simulink model "ANN_and_Fuzzy_NCD"  (R2024a)
settings: Solver=ode23  StartTime=0.0  StopTime=200  RelTol=1e-8  EnableMultiTasking=on
model workspace (MAT data in the model file):
  targetSettings3.name = 'mapminmax'
  targetSettings3.xrows = 1
  targetSettings3.xmax = 42104.0119289
  targetSettings3.xmin = -1.27777923922
  targetSettings3.xrange = 42105.2897081
  targetSettings3.yrows = 1
  targetSettings3.ymax = 1
  targetSettings3.ymin = -1
  targetSettings3.yrange = 2
  targetSettings3.gain = 4.74999700481e-05
  targetSettings3.xoffset = -1.27777923922
  targetSettings3.no_change = 0
values from neighbouring files (symbols this model uses):
  I = in1'    [ann_training.m]
  T = out1'    [ann_training.m]
undefined symbols (not defined in the file or in its folder): B, DL, DQ, m, M, magnitude, rg, W, xb, xg, Xudot, yb, yg, Yvdot, zb, zg, Zwdot
libraries: neural x270, simulink x28, fuzblock x3
(part 1 of 12)
settings Model: Creator=hoang  LastModifiedBy=Long
settings SolverCC: ZeroCrossAlgorithm=Adaptive
settings DataIOCC: LimitDataPoints=on  SaveFormat=Array  SignalLoggingSaveFormat=ModelDataLogs  ReturnWorkspaceOutputs=off
settings OptimizationCC: InitFltsAndDblsToZero=on  LifeSpan=inf
settings DebuggingCC: SaveWithParameterizedLinksMsg=none  UnderspecifiedInitializationDetection=Classic  MergeDetectMultiDrivingBlocksExec=none  SignalResolutionControl=TryResolveAllWithWarning  IgnoredZcDiagnostic=none  SolverPrmCheckMsg=warning  MultiTaskDSMMsg=warning  MultiTaskCondExecSysMsg=none  UnconnectedInputMsg=warning  UnconnectedOutputMsg=warning  UnconnectedLineMsg=warning  SFUnexpectedBacktrackingDiag=warning  SFNoUnconditionalDefaultTransitionDiag=warning  SFExecutionAtInitializationDiag=none  ArithmeticOperatorsInVariantConditions=warning
settings HardwareCC: ProdBitPerPointer=32  ProdBitPerSizeT=32  ProdBitPerPtrDiffT=32  ProdLargestAtomicFloat=None  ProdIntDivRoundTo=Undefined  ProdEndianess=Unspecified  ProdWordSize=32  ProdHWDeviceType=32-bit Generic
settings ModelReferenceCC: EnableRefExpFcnMdlSchedulingChecks=on  PropagateSignalLabelsOutOfModel=off
settings RTWCC: GPUComputeCapability=3.5  DLArmComputeVersion=19.05
settings CodeAppCC: StateflowObjectComments=on
settings GRTTargetCC: TargetFcnLib=ansi_tfl_tmw.mat  TargetLangStandard=C89/C90 (ANSI)  CombineOutputUpdateFcns=off  GRTInterface=on
settings ConfigComp: CovMetricSettings=dw  CovSaveCumulativeToWorkspaceVar=on  CovSaveSingleToWorkspaceVar=on

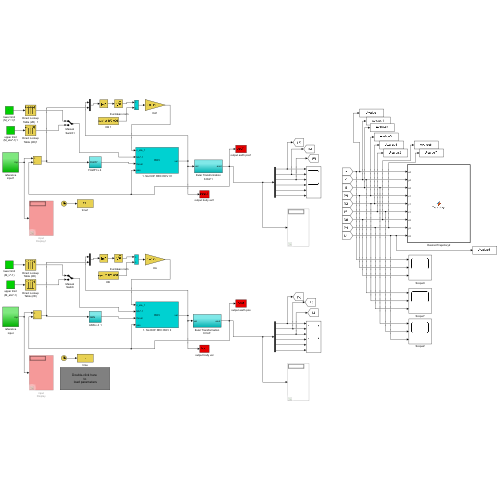
[thumbnail: Simulink's stored preview of the top-level diagram]
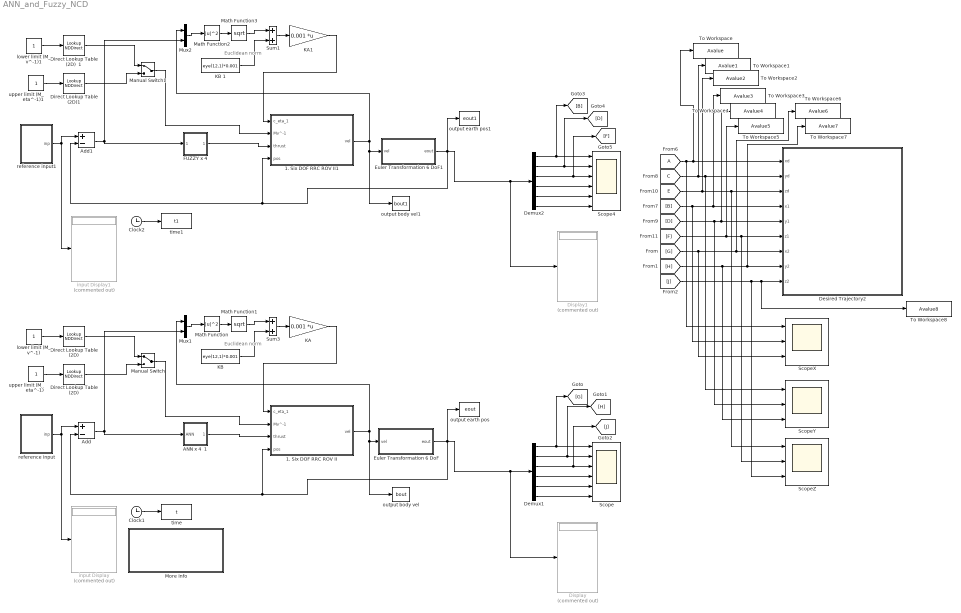
== system ANN_and_Fuzzy_NCD ==
  note: Euclidean norm
  note: Euclidean norm
  " ANN x 4  1" : Subsystem  AncestorBlock=|
      | rov_design_analysis/ROV Controller
      | Design
      | Applications/8. PID x 4
  " FUZZY x 4  " : Subsystem  AncestorBlock=|
      | rov_design_analysis/ROV Controller
      | Design
      | Applications/8. PID x 4
  1. Six DOF RRC ROV II : Subsystem  AncestorBlock=rov_design_analysis/ROV Models/1. Six DOF RRC ROV II
      mask Display: disp('ROV')
  1. Six DOF RRC ROV II1 : Subsystem  AncestorBlock=rov_design_analysis/ROV Models/1. Six DOF RRC ROV II
      mask Display: disp('ROV')
  Add : Sum  Inputs=+-
  Add1 : Sum  Inputs=+-
  Clock1 : Clock
  Clock2 : Clock
  Demux1 : Demux  Outputs=6
  Demux2 : Demux  Outputs=6
  Desired Trajectory2 : MATLAB Function  TreatAsAtomicUnit=on
  Direct Lookup Table (2D) : LookupNDDirect  InputsSelectThisObjectFromTable=Vector  Table=[0:0.1:1;0:0.1:1;0:0.1:1; 0:0.1:1 ; 0:0.1:1 ;0:0.1:1]*0.0001
  "Direct Lookup Table (2D)  " : LookupNDDirect  InputsSelectThisObjectFromTable=Vector  Table=-[0:0.1:1;0:0.1:1;0:0.1:1; 0:0.1:1 ; 0:0.1:1 ;0:0.1:1]*0.001
  Direct Lookup Table (2D)  1 : LookupNDDirect  InputsSelectThisObjectFromTable=Vector  Table=-[0:0.1:1;0:0.1:1;0:0.1:1; 0:0.1:1 ; 0:0.1:1 ;0:0.1:1]*0.001
  Direct Lookup Table (2D)1 : LookupNDDirect  InputsSelectThisObjectFromTable=Vector  Table=[0:0.1:1;0:0.1:1;0:0.1:1; 0:0.1:1 ; 0:0.1:1 ;0:0.1:1]*0.0001
  Display : Display  Commented=on
  Display1 : Display  Commented=on
  Euler Transformation 6 DoF : Subsystem  AncestorBlock=rov_design_analysis/Utilities/Euler Transformation 6 DoF
  Euler Transformation 6 DoF1 : Subsystem  AncestorBlock=rov_design_analysis/Utilities/Euler Transformation 6 DoF
  From6 : From  TagVisibility=global
  KA : Gain  Gain=0.001  Multiplication=Matrix(K*u)  SaturateOnIntegerOverflow=on  OutDataTypeStr=Inherit: Same as input  ParamDataTypeStr=Inherit: Same as input
  KA1 : Gain  Gain=0.001  Multiplication=Matrix(K*u)  SaturateOnIntegerOverflow=on  OutDataTypeStr=Inherit: Same as input  ParamDataTypeStr=Inherit: Same as input
  "KB " : Constant  Value=eye(12,1)*0.001
  KB 1 : Constant  Value=eye(12,1)*0.001
  Manual Switch : ManualSwitch
  Manual Switch1 : ManualSwitch
  Math Function : Math  Operator=magnitude^2  SignedPower=on
  Math Function1 : Math  Operator=sqrt  SignedPower=on
  Math Function2 : Math  Operator=magnitude^2  SignedPower=on
  Math Function3 : Math  Operator=sqrt  SignedPower=on
  More Info : Subsystem
      settings: OpenFcn=|
      | cd c:\Matlab7\toolbox\rov_design_analysis\\mat_file ;
      | load rrcrovf;
      | kp1=11;ki1=2;kd1=1; kp2=11;ki2=4;kd2=1;kp3=9;ki3=1;kd3=2;kp4=1;ki4=2;kd4=1;
      mask Display: disp('Double-click here \n to \n load parameters')
  Mux1 : Mux  Inputs=2
  Mux2 : Mux  Inputs=2
  Scope : Scope  NumInputPorts=6
  Scope4 : Scope  NumInputPorts=6
  ScopeX : Scope  NumInputPorts=3
  ScopeY : Scope  NumInputPorts=3
  ScopeZ : Scope  NumInputPorts=3
  Sum1 : Sum  OutDataTypeStr=double  SaturateOnIntegerOverflow=on
  Sum3 : Sum  OutDataTypeStr=double  SaturateOnIntegerOverflow=on
  To Workspace : ToWorkspace  VariableName=Avalue  SampleTime=-1
  To Workspace1 : ToWorkspace  VariableName=Avalue1  SampleTime=-1
  To Workspace2 : ToWorkspace  VariableName=Avalue2  SampleTime=-1
  To Workspace3 : ToWorkspace  VariableName=Avalue3  SampleTime=-1
  To Workspace4 : ToWorkspace  VariableName=Avalue4  SampleTime=-1
  To Workspace5 : ToWorkspace  VariableName=Avalue5  SampleTime=-1
  To Workspace6 : ToWorkspace  VariableName=Avalue6  SampleTime=-1
  To Workspace7 : ToWorkspace  VariableName=Avalue7  SampleTime=-1
  To Workspace8 : ToWorkspace  VariableName=Avalue8  SampleTime=-1
  input Display : Display  Commented=on
  input Display1 : Display  Commented=on
  lower limit (M_v^-1) : Constant
  lower limit (M_v^-1)1 : Constant
  output body vel : ToWorkspace  VariableName=bout  SampleTime=1
  output body vel1 : ToWorkspace  VariableName=bout1  SampleTime=1
  output earth pos : ToWorkspace  VariableName=eout  SampleTime=1
  output earth pos1 : ToWorkspace  VariableName=eout1  SampleTime=1
  reference input : Subsystem  AncestorBlock=|
      | rov_design_analysis/Scope
      | Utilities/pipe tracking
      | profile 
      | (Manual)
  reference input1 : Subsystem  AncestorBlock=|
      | rov_design_analysis/Scope
      | Utilities/pipe tracking
      | profile 
      | (Manual)
  time : ToWorkspace  VariableName=t  SampleTime=1
  time1 : ToWorkspace  VariableName=t1  SampleTime=1
  upper limit (M_eta^-1) : Constant
  upper limit (M_eta^-1)1 : Constant
  wires:
  Euler Transformation 6 DoF/1(eout) -> output earth pos/1, Add/2, 1. Six DOF RRC ROV II/4("pos "), Display/1, Demux1/1
  Clock1/1 -> time/1
  Add/1 -> " ANN x 4  1"/1(ANN), Mux1/2
  reference input/1(inp) -> Add/1, input Display/1
  1. Six DOF RRC ROV II/1(vel) -> output body vel/1, Euler Transformation 6 DoF/1(vel), Mux1/1
  upper limit (M_eta^-1)/1 -> Direct Lookup Table (2D)/1
  lower limit (M_v^-1)/1 -> "Direct Lookup Table (2D)  "/1
  "Direct Lookup Table (2D)  "/1 -> Manual Switch/1
  Manual Switch/1 -> 1. Six DOF RRC ROV II/2(Mv^-1)
  Direct Lookup Table (2D)/1 -> Manual Switch/2
  Sum3/1 -> KA/1
  "KB "/1 -> Sum3/2
  Mux1/1 -> Math Function/1
  Math Function/1 -> Math Function1/1
  Math Function1/1 -> Sum3/1
  KA/1 -> 1. Six DOF RRC ROV II/1(c_eta_1)
  Demux1/1 -> [G], Scope/1
  Demux1/2 -> [H], Scope/2
  Demux1/3 -> [J], Scope/3
  Demux1/6 -> Scope/6
  Demux1/5 -> Scope/5
  Demux1/4 -> Scope/4
  KB 1/1 -> Sum1/2
  Demux2/2 -> [D], Scope4/2
  [C] -> To Workspace1/1, ScopeY/1, Desired Trajectory2/2(yd)
  Sum1/1 -> KA1/1
  [D] -> ScopeY/2, To Workspace4/1, Desired Trajectory2/5(y1)
  lower limit (M_v^-1)1/1 -> Direct Lookup Table (2D)  1/1
  Manual Switch1/1 -> 1. Six DOF RRC ROV II1/2(Mv^-1)
  [F] -> To Workspace5/1, ScopeZ/2, Desired Trajectory2/6(z1)
  KA1/1 -> 1. Six DOF RRC ROV II1/1(c_eta_1)
  1. Six DOF RRC ROV II1/1(vel) -> output body vel1/1, Euler Transformation 6 DoF1/1(vel), Mux2/1
  From6/1 -> ScopeX/1, To Workspace/1, Desired Trajectory2/1(xd)
  Add1/1 -> Mux2/2, " FUZZY x 4  "/1(FUZZY)
  Demux2/4 -> Scope4/4
  Demux2/3 -> [F], Scope4/3
  Demux2/5 -> Scope4/5
  Demux2/6 -> Scope4/6
  Direct Lookup Table (2D)1/1 -> Manual Switch1/2
  Demux2/1 -> [B], Scope4/1
  reference input1/1(inp) -> Add1/1, input Display1/1
  Euler Transformation 6 DoF1/1(eout) -> output earth pos1/1, Add1/2, 1. Six DOF RRC ROV II1/4("pos "), Display1/1, Demux2/1
  Mux2/1 -> Math Function2/1
  Math Function2/1 -> Math Function3/1
  Math Function3/1 -> Sum1/1
  Direct Lookup Table (2D)  1/1 -> Manual Switch1/1
  upper limit (M_eta^-1)1/1 -> Direct Lookup Table (2D)1/1
  Clock2/1 -> time1/1
  [B] -> ScopeX/2, To Workspace3/1, Desired Trajectory2/4(x1)
  [E] -> ScopeZ/1, Desired Trajectory2/3(zd), To Workspace2/1
  " FUZZY x 4  "/1(" ") -> 1. Six DOF RRC ROV II1/3("thrust ")
  [G] -> ScopeX/3, To Workspace6/1, Desired Trajectory2/7(x2)
  [H] -> ScopeY/3, To Workspace7/1, Desired Trajectory2/8(y2)
  [J] -> ScopeZ/3, To Workspace8/1, Desired Trajectory2/9(z2)
  " ANN x 4  1"/1(" ") -> 1. Six DOF RRC ROV II/3("thrust ")

== system ANN_and_Fuzzy_NCD/ ANN x 4  1 ==
  ANN : Inport
  ANN X : Subsystem  Commented=on
      mask help: Feed-Forward Neural Network
      mask Display: e = 0.06;c1 = [120 150 230]/255;c2 = ([120 150 230]+0)/383;c3 = ([120 150 230]+128)/383;patch([0 1 1 0],[0 0 1 1],c1);patch([0 1 1 1-e 1-e 0+e],[0 0 1 1-e 0+e 0+e],c2);patch([0 0 1 1-e 0+e 0+e],[0 1 1 1-e 1-e 0+e],c3);plot([0 1 1 0 0],[0 0 1 1 0]);fprintf('NNET');port_label('input',1,' Input');port_label('output',1,'Output ');
  ANN Y : Subsystem  Commented=on
      mask help: Feed-Forward Neural Network
      mask Display: e = 0.06;c1 = [120 150 230]/255;c2 = ([120 150 230]+0)/383;c3 = ([120 150 230]+128)/383;patch([0 1 1 0],[0 0 1 1],c1);patch([0 1 1 1-e 1-e 0+e],[0 0 1 1-e 0+e 0+e],c2);patch([0 0 1 1-e 0+e 0+e],[0 1 1 1-e 1-e 0+e],c3);plot([0 1 1 0 0],[0 0 1 1 0]);fprintf('NNET');port_label('input',1,' Input');port_label('output',1,'Output ');
  ANN Z : Subsystem  Commented=on
      mask help: Feed-Forward Neural Network
      mask Display: e = 0.06;c1 = [120 150 230]/255;c2 = ([120 150 230]+0)/383;c3 = ([120 150 230]+128)/383;patch([0 1 1 0],[0 0 1 1],c1);patch([0 1 1 1-e 1-e 0+e],[0 0 1 1-e 0+e 0+e],c2);patch([0 0 1 1-e 0+e 0+e],[0 1 1 1-e 1-e 0+e],c3);plot([0 1 1 0 0],[0 0 1 1 0]);fprintf('NNET');port_label('input',1,' Input');port_label('output',1,'Output ');
  Demux1 : Demux  Outputs=6
      settings: DisplayOption=none
  Mux2 : Mux  Inputs=6
  Subsystem : Subsystem
  Subsystem1 : Subsystem
  Subsystem2 : Subsystem
  X_1 : Subsystem
      mask help: Feed-Forward Neural Network
      mask Display: e = 0.06;c1 = [120 150 230]/255;c2 = ([120 150 230]+0)/383;c3 = ([120 150 230]+128)/383;patch([0 1 1 0],[0 0 1 1],c1);patch([0 1 1 1-e 1-e 0+e],[0 0 1 1-e 0+e 0+e],c2);patch([0 0 1 1-e 0+e 0+e],[0 1 1 1-e 1-e 0+e],c3);plot([0 1 1 0 0],[0 0 1 1 0]);fprintf('NNET');port_label('input',1,' Input');port_label('output',1,'Output ');
  Y_1 : Subsystem
      mask help: Feed-Forward Neural Network
      mask Display: e = 0.06;c1 = [120 150 230]/255;c2 = ([120 150 230]+0)/383;c3 = ([120 150 230]+128)/383;patch([0 1 1 0],[0 0 1 1],c1);patch([0 1 1 1-e 1-e 0+e],[0 0 1 1-e 0+e 0+e],c2);patch([0 0 1 1-e 0+e 0+e],[0 1 1 1-e 1-e 0+e],c3);plot([0 1 1 0 0],[0 0 1 1 0]);fprintf('NNET');port_label('input',1,' Input');port_label('output',1,'Output ');
  Z_1 : Subsystem
      mask help: Feed-Forward Neural Network
      mask Display: e = 0.06;c1 = [120 150 230]/255;c2 = ([120 150 230]+0)/383;c3 = ([120 150 230]+128)/383;patch([0 1 1 0],[0 0 1 1],c1);patch([0 1 1 1-e 1-e 0+e],[0 0 1 1-e 0+e 0+e],c2);patch([0 0 1 1-e 0+e 0+e],[0 1 1 1-e 1-e 0+e],c3);plot([0 1 1 0 0],[0 0 1 1 0]);fprintf('NNET');port_label('input',1,' Input');port_label('output',1,'Output ');
  " " : Outport
  wires:
  Demux1/4 -> Mux2/4
  Demux1/5 -> Mux2/5
  Demux1/6 -> Mux2/6
  Demux1/2 -> Subsystem1/1(In1)
  Demux1/3 -> Subsystem2/1(In1)
  ANN/1 -> Demux1/1
  Mux2/1 -> " "/1
  Demux1/1 -> Subsystem/1(In1)
  Subsystem/1(Out1) -> X_1/1(Input)
  Subsystem1/1(Out1) -> Y_1/1(Input)
  Subsystem2/1(Out1) -> Z_1/1(Input)
  X_1/1(Output) -> Mux2/1
  Z_1/1(Output) -> Mux2/3
  Y_1/1(Output) -> Mux2/2

== system ANN_and_Fuzzy_NCD/ FUZZY x 4   ==
  FUZZY : Inport
  Demux1 : Demux  Outputs=6
      settings: DisplayOption=none
  Mux2 : Mux  Inputs=6
  Subsystem1 : Subsystem
  Subsystem5 : Subsystem
  Subsystem6 : Subsystem
  " " : Outport
  wires:
  Demux1/1 -> Subsystem1/1(Error)
  Demux1/4 -> Mux2/4
  Demux1/5 -> Mux2/5
  Subsystem1/1(Output) -> Mux2/1
  Subsystem6/1(Output) -> Mux2/3
  Demux1/2 -> Subsystem5/1(Error)
  Subsystem5/1(Output) -> Mux2/2
  Demux1/3 -> Subsystem6/1(Error)
  FUZZY/1 -> Demux1/1
  Mux2/1 -> " "/1
  Demux1/6 -> Mux2/6

== system ANN_and_Fuzzy_NCD/1. Six DOF RRC ROV II ==
  c_eta_1 : Inport
  Mv^-1 : Inport  Port=2
  "thrust " : Inport  Port=3
  "pos " : Inport  Port=4
  Centripetal & Coriolis : Subsystem
      mask Display: disp('Coriolis \n& Centrpetal \nMatrix')
  Demux : Demux  Outputs=2
  Hydrodynamic Damping : Subsystem
      mask Display: disp('Hydrodynamic \nDamping')
  Integrator1 : Integrator  UpperSaturationLimit=5  LowerSaturationLimit=1
  Mass Inertia Matrix : Subsystem
      mask Display: disp('Inverse Mass \n Inertia \n Matrix')
  Pseudo Inverse : Gain  Gain=pinv(T)  Multiplication=Matrix(K*u)  SaturateOnIntegerOverflow=on  OutDataTypeStr=Inherit: Same as input  ParamDataTypeStr=Inherit: Same as input
  Restoring Forces : Subsystem
      mask Display: disp('Restoring\nForce')
  Sum1 : Sum  Inputs=+---  OutDataTypeStr=double  SaturateOnIntegerOverflow=on
  Sum2 : Sum  OutDataTypeStr=double  SaturateOnIntegerOverflow=on
  Sum3 : Sum  OutDataTypeStr=double  SaturateOnIntegerOverflow=on
  Sum4 : Sum  OutDataTypeStr=double  SaturateOnIntegerOverflow=on
  Thruster Configuration Matrix (n X n) : Subsystem  AncestorBlock=|  mask(Thruster Configuration Matrix){T=T}
      | rov_design_analysis/ROV
      | Models/4.  Thruster Configuration Matrix
      | (n X n)
      mask prompts: T "Insert Thruster Configuration Matrix"
      mask help: Provide the thruster configuration matrix using summation of forces and moment about the vehicle's C.G.
      mask Display: disp('Thruster \n Configuration')
  vel : Outport
  wires:
  Sum1/1 -> Mass Inertia Matrix/1(In)
  "pos "/1 -> Restoring Forces/1(pos)
  Restoring Forces/1(gravitational force) -> Sum1/2
  "thrust "/1 -> Pseudo Inverse/1
  Pseudo Inverse/1 -> Thruster Configuration Matrix (n X n)/1(In1)
  Sum2/1 -> Integrator1/1
  Mass Inertia Matrix/1(Out) -> Sum2/2
  Mv^-1/1 -> Sum2/1
  Centripetal & Coriolis/1(force) -> Sum3/2
  Sum3/1 -> Sum1/4
  Sum4/1 -> Sum1/3
  Hydrodynamic Damping/1(damping force) -> Sum4/2
  c_eta_1/1 -> Demux/1
  Demux/2 -> Sum4/1
  Demux/1 -> Sum3/1
  Integrator1/1 -> vel/1, Centripetal & Coriolis/1(vel), Hydrodynamic Damping/1(vel)
  Thruster Configuration Matrix (n X n)/1(Out1) -> Sum1/1

== system ANN_and_Fuzzy_NCD/1. Six DOF RRC ROV II1 ==
  c_eta_1 : Inport
  Mv^-1 : Inport  Port=2
  "thrust " : Inport  Port=3
  "pos " : Inport  Port=4
  Centripetal & Coriolis : Subsystem
      mask Display: disp('Coriolis \n& Centrpetal \nMatrix')
  Demux : Demux  Outputs=2
  Hydrodynamic Damping : Subsystem
      mask Display: disp('Hydrodynamic \nDamping')
  Integrator1 : Integrator  UpperSaturationLimit=5  LowerSaturationLimit=1
  Mass Inertia Matrix : Subsystem
      mask Display: disp('Inverse Mass \n Inertia \n Matrix')
  Pseudo Inverse : Gain  Gain=pinv(T)  Multiplication=Matrix(K*u)  SaturateOnIntegerOverflow=on  OutDataTypeStr=Inherit: Same as input  ParamDataTypeStr=Inherit: Same as input
  Restoring Forces : Subsystem
      mask Display: disp('Restoring\nForce')
  Sum1 : Sum  Inputs=+---  OutDataTypeStr=double  SaturateOnIntegerOverflow=on
  Sum2 : Sum  OutDataTypeStr=double  SaturateOnIntegerOverflow=on
  Sum3 : Sum  OutDataTypeStr=double  SaturateOnIntegerOverflow=on
  Sum4 : Sum  OutDataTypeStr=double  SaturateOnIntegerOverflow=on
  Thruster Configuration Matrix (n X n) : Subsystem  AncestorBlock=|  mask(Thruster Configuration Matrix){T=T}
      | rov_design_analysis/ROV
      | Models/4.  Thruster Configuration Matrix
      | (n X n)
      mask prompts: T "Insert Thruster Configuration Matrix"
      mask help: Provide the thruster configuration matrix using summation of forces and moment about the vehicle's C.G.
      mask Display: disp('Thruster \n Configuration')
  vel : Outport
  wires:
  Sum1/1 -> Mass Inertia Matrix/1(In)
  "pos "/1 -> Restoring Forces/1(pos)
  Restoring Forces/1(gravitational force) -> Sum1/2
  Thruster Configuration Matrix (n X n)/1(Out1) -> Sum1/1
  "thrust "/1 -> Pseudo Inverse/1
  Pseudo Inverse/1 -> Thruster Configuration Matrix (n X n)/1(In1)
  Sum2/1 -> Integrator1/1
  Integrator1/1 -> vel/1, Centripetal & Coriolis/1(vel), Hydrodynamic Damping/1(vel)
  Mass Inertia Matrix/1(Out) -> Sum2/2
  Mv^-1/1 -> Sum2/1
  Centripetal & Coriolis/1(force) -> Sum3/2
  Sum3/1 -> Sum1/4
  Sum4/1 -> Sum1/3
  Hydrodynamic Damping/1(damping force) -> Sum4/2
  c_eta_1/1 -> Demux/1
  Demux/2 -> Sum4/1
  Demux/1 -> Sum3/1

== system ANN_and_Fuzzy_NCD/Euler Transformation 6 DoF ==
  vel : Inport
  Demux : Demux  Outputs=2
      settings: DisplayOption=none
  Demux1 : Demux  Outputs=2
      settings: DisplayOption=none
  Environment Impact2 : Subsystem
  Intregrator2 : Integrator
  Mux1 : Mux  Inputs=2
  Sum : Sum  Inputs=|++
  Terminator : Terminator
  Transformation matrix R : Subsystem
      mask Display: disp('Transformation R')
  Transformation matrix T : Subsystem
      mask Display: disp('Transformation T')
  eout : Outport  InitialOutput=0
  wires:
  Mux1/1 -> Intregrator2/1
  Intregrator2/1 -> Sum/2, Demux1/1
  Demux/2 -> Transformation matrix R/1(angular body velocity)
  Demux/1 -> Transformation matrix T/1(translational body velocity)
  vel/1 -> Demux/1
  Demux1/2 -> Transformation matrix T/2(angular position), Transformation matrix R/2(angular position)
  Transformation matrix R/1(angular earth velocity) -> Mux1/2
  Transformation matrix T/1(translational earth velocity) -> Mux1/1
  Demux1/1 -> Terminator/1
  Sum/1 -> eout/1
  Environment Impact2/1(F_current) -> Sum/1

== system ANN_and_Fuzzy_NCD/Euler Transformation 6 DoF1 ==
  vel : Inport
  Demux : Demux  Outputs=2
      settings: DisplayOption=none
  Demux1 : Demux  Outputs=2
      settings: DisplayOption=none
  Environment Impact2 : Subsystem
  Intregrator2 : Integrator
  Mux1 : Mux  Inputs=2
  Sum : Sum  Inputs=|++
  Terminator : Terminator
  Transformation matrix R : Subsystem
      mask Display: disp('Transformation R')
  Transformation matrix T : Subsystem
      mask Display: disp('Transformation T')
  eout : Outport  InitialOutput=0
  wires:
  Mux1/1 -> Intregrator2/1
  Intregrator2/1 -> Sum/2, Demux1/1
  Demux/2 -> Transformation matrix R/1(angular body velocity)
  Demux/1 -> Transformation matrix T/1(translational body velocity)
  vel/1 -> Demux/1
  Demux1/2 -> Transformation matrix T/2(angular position), Transformation matrix R/2(angular position)
  Transformation matrix R/1(angular earth velocity) -> Mux1/2
  Transformation matrix T/1(translational earth velocity) -> Mux1/1
  Demux1/1 -> Terminator/1
  Sum/1 -> eout/1
  Environment Impact2/1(F_current) -> Sum/1

== system ANN_and_Fuzzy_NCD/More Info ==

== system ANN_and_Fuzzy_NCD/reference input ==
  Goto : Goto  TagVisibility=global
  Ground : Ground
  Mux : Mux  Inputs=6
  Repeating Sequence Stair13 : simulink/Sources/Repeating Sequence Stair  OutValues="[0 1 2 3 4 5 6 7 8 9 10 11 12 13 14 15 16 17 18 19 20 20 20 20 20 20 20 20 20 20 20 20 20 20 20 20 20 20 20 20 20 20 20 20 20 20 20 20 20 20 20 20 20 20 20 20 20 20 20 20 20 20 20 20 20 20 20 20 20 20 20 20 20 20 20 20 20 20 20 20 20 20 20 20 20 20 20 20 20 20 20 20 20 20 20 20   ].'"  tsamp=2.5  OutMin=[]  OutMax=[]  OutDataTypeStr=double  OutputDataTypeScalingMode=double  OutDataType=fixdt(0,8)  ConRadixGroup=Best Precision: Vector-wise  OutScaling=2^-12
  Repeating Sequence Stair14 : simulink/Sources/Repeating Sequence Stair  OutValues="[0 0.5 1 1.5 2 2.5 3 3.5 4 4.5 5 5.5 6 6.5 7 7.5 8 8.5 9 9.5 10 10 10 10 10 10 10 10 10 10 10 10 10 10 10 10 10 10 10 10 10 10 10 10 10 10 10 10 10 10 10 10 10 10 10 10 10 10 10 10 10 10 10 10 10 10 10 10 10 10 10 10 10 10 10 10 10 10 10 10 10 10 10 10 10 10 10 10 10 10 10 10 10 10 10 10 10 10 10 10 10 10 10 10 10 10 10 10 10 10 10 10 10 10 10 10 10 10 10 10 10 10 10 10 10 10 10 10 10 10 10 10 10 10 10 10 10 10 10 10 10 10 10 10 10 10 10 10 10 10 10 10 10 10 10 10 10 10 10 10 10 10 10 10 10 10 10 10 10 10 10 10 10     ].'"  tsamp=2.5  OutMin=[]  OutMax=[]  OutDataTypeStr=double  OutputDataTypeScalingMode=double  OutDataType=fixdt(0,8)  ConRadixGroup=Best Precision: Vector-wise  OutScaling=2^-12
  Repeating Sequence Stair15 : simulink/Sources/Repeating Sequence Stair  OutValues="[0 1 2 3 4 5 6 7 8 9 10 11 12 13 14 15 16 17 18 19 20 20 20 20 20 20 20 20 20 20 20 20 20 20 20 20 20 20 20 20 20 20 20 20 20 20 20 20 20 20 20 20 20 20 20 20 20 20 20 20 20 20 20 20 20 20 20 20 20 20 20 20 20 20 20 20 20 20 20 20 20 20 20 20 20    ].'"  tsamp=2.5  OutMin=[]  OutMax=[]  OutDataTypeStr=double  OutputDataTypeScalingMode=double  OutDataType=fixdt(0,8)  ConRadixGroup=Best Precision: Vector-wise  OutScaling=2^-12
  Repeating Sequence Stair3 : simulink/Sources/Repeating Sequence Stair  OutValues="[0 0 0 0 0 0 0 0 0 0 0 0 0 0 0 0 0 0 0 0 0 0 0 0 0 0 0 0 0 0 0 0 0 0 0 0 0 0 0 0 0 0 0 0 0 0 0 0 0 0 0 0 0 0 0 0 0 0 0 0 0 0 0 0 0 0 0 0 0 0 0 0 0 0 0 0 0 0 0 0 0 0 0 0 0 0 0 0 0 0 0 0 0 0 0 0 0 0 0 0 0 0 0 0 0 0 0 0 0 0 0 0 0 0 0 0 0 0 0 0 0 0 0 0 0 0 0 0 0 0 0 0 0 0 0 0 0 0 0 0 0 0 0 0 0 0 0 0 0 0 0 0 0 0 0 0 0 0 0 0 0 0 0 0 0  ].'"  tsamp=2.5  OutMin=[]  OutMax=[]  OutDataTypeStr=double  OutputDataTypeScalingMode=double  OutDataType=fixdt(0,8)  ConRadixGroup=Best Precision: Vector-wise  OutScaling=2^-12
  Repeating Sequence Stair4 : simulink/Sources/Repeating Sequence Stair  Commented=on  OutValues="[0 1 2 3 4 5 6 7 8 9 10 10 10 10 10 10 10 10 10 10 10 10 10 10 10 10 10 10 10 10 10 11 12 13 14 15 16 17 18 19 20 20 20 20 20 20 20 20 20 20 20 19 18 17 16 15 14 13 12 11 10 10 10 10 10 10 10 10 10 10 10 10 10 10 10 10 10 10 10 10 10 10 10 10 10 10 10 10 10 10 10 10 10 10 10 10 10 10 10 10  ].'"  tsamp=2.5  OutMin=[]  OutMax=[]  OutDataTypeStr=double  OutputDataTypeScalingMode=double  OutDataType=fixdt(0,8)  ConRadixGroup=Best Precision: Vector-wise  OutScaling=2^-12
  Repeating Sequence Stair5 : simulink/Sources/Repeating Sequence Stair  Commented=on  OutValues=[0 0 0 0 0 0 0 0 0 0 0 0.5 1 1.5 2 2.5 3 3.5 4 4.5 5 5 5 5 5 5 5 5 5 5 5 5 5 5 5 5 5 5 5 5 5 5.5 6 6.5 7 7.5 8 8.5 9 9.5 10 10 10 10 10 10 10 10 10 10 10 10 10 10 10 10 10 10 10 10 10 10 10 10 10 10 10 10 10 10 10 10 10 10 10 10 10 10 10 10 10 10 10 10 10 10 10 10 10 10 10 10 10 10 10 10 10 10 10 10 10 10 10 10 10 10 10 10 10 10 10 10 10 10 10 10].'  tsamp=2.5  OutMin=[]  OutMax=[]  OutDataTypeStr=double  OutputDataTypeScalingMode=double  OutDataType=fixdt(0,8)  ConRadixGroup=Best Precision: Vector-wise  OutScaling=2^-12
  Repeating Sequence Stair6 : simulink/Sources/Repeating Sequence Stair  Commented=on  OutValues="[0 0 0 0 0 0 0 0 0 0 0 0 0 0 0 0 0 0 0 0 0 1 2 3 4 5 6 7 8 9 10 10 10 10 10 10 10 10 10 10 10 10 10 10 10 10 10 10 10 10 10 10 10 10 10 10 10 10 10 10 10 10 10 10 10 10 10 10 10 10 10 10 10 10 10 10 10 10 10 10 10 10 10 10 10 10 10 10 10 10 10 10 10 10 10 10 10 10 10 10 10 10 10 10 10 10 10 10 10 10 10 10 10 10 10 10 10 10 10 10 10 10 10 10 10 10 10 10 10 10 10 10 10 10  ].'"  tsamp=2.5  OutMin=[]  OutMax=[]  OutDataTypeStr=double  OutputDataTypeScalingMode=double  OutDataType=fixdt(0,8)  ConRadixGroup=Best Precision: Vector-wise  OutScaling=2^-12
  inp : Outport
  tag scope: C=global, E=global
  wires:
  Mux/1 -> inp/1
  Ground/1 -> Mux/4, Mux/5
  Repeating Sequence Stair3/1 -> Mux/6
  Repeating Sequence Stair13/1 -> Goto/1, Mux/1
  Repeating Sequence Stair14/1 -> [C], Mux/2
  Repeating Sequence Stair15/1 -> [E], Mux/3

== system ANN_and_Fuzzy_NCD/reference input1 ==
  Ground : Ground
  Mux : Mux  Inputs=6
  Repeating Sequence Stair13 : simulink/Sources/Repeating Sequence Stair  OutValues="[0 1 2 3 4 5 6 7 8 9 10 11 12 13 14 15 16 17 18 19 20 20 20 20 20 20 20 20 20 20 20 20 20 20 20 20 20 20 20 20 20 20 20 20 20 20 20 20 20 20 20 20 20 20 20 20 20 20 20 20 20 20 20 20 20 20 20 20 20 20 20 20 20 20 20 20 20 20 20 20 20 20 20 20 20 20 20 20 20 20 20 20 20 20 20 20   ].'"  tsamp=2.5  OutMin=[]  OutMax=[]  OutDataTypeStr=double  OutputDataTypeScalingMode=double  OutDataType=fixdt(0,8)  ConRadixGroup=Best Precision: Vector-wise  OutScaling=2^-12
  Repeating Sequence Stair14 : simulink/Sources/Repeating Sequence Stair  OutValues="[0 0.5 1 1.5 2 2.5 3 3.5 4 4.5 5 5.5 6 6.5 7 7.5 8 8.5 9 9.5 10 10 10 10 10 10 10 10 10 10 10 10 10 10 10 10 10 10 10 10 10 10 10 10 10 10 10 10 10 10 10 10 10 10 10 10 10 10 10 10 10 10 10 10 10 10 10 10 10 10 10 10 10 10 10 10 10 10 10 10 10 10 10 10 10 10 10 10 10 10 10 10 10 10 10 10 10 10 10 10 10 10 10 10 10 10 10 10 10 10 10 10 10 10 10 10 10 10 10 10 10 10 10 10 10 10 10 10 10 10 10 10 10 10 10 10 10 10 10 10 10 10 10 10 10 10 10 10 10 10 10 10 10 10 10 10 10 10 10 10 10 10 10 10 10 10 10 10 10 10 10 10 10     ].'"  tsamp=2.5  OutMin=[]  OutMax=[]  OutDataTypeStr=double  OutputDataTypeScalingMode=double  OutDataType=fixdt(0,8)  ConRadixGroup=Best Precision: Vector-wise  OutScaling=2^-12
  Repeating Sequence Stair15 : simulink/Sources/Repeating Sequence Stair  OutValues="[0 1 2 3 4 5 6 7 8 9 10 11 12 13 14 15 16 17 18 19 20 20 20 20 20 20 20 20 20 20 20 20 20 20 20 20 20 20 20 20 20 20 20 20 20 20 20 20 20 20 20 20 20 20 20 20 20 20 20 20 20 20 20 20 20 20 20 20 20 20 20 20 20 20 20 20 20 20 20 20 20 20 20 20 20    ].'"  tsamp=2.5  OutMin=[]  OutMax=[]  OutDataTypeStr=double  OutputDataTypeScalingMode=double  OutDataType=fixdt(0,8)  ConRadixGroup=Best Precision: Vector-wise  OutScaling=2^-12
  Repeating Sequence Stair3 : simulink/Sources/Repeating Sequence Stair  OutValues="[0 0 0 0 0 0 0 0 0 0 0 0 0 0 0 0 0 0 0 0 0 0 0 0 0 0 0 0 0 0 0 0 0 0 0 0 0 0 0 0 0 0 0 0 0 0 0 0 0 0 0 0 0 0 0 0 0 0 0 0 0 0 0 0 0 0 0 0 0 0 0 0 0 0 0 0 0 0 0 0 0 0 0 0 0 0 0 0 0 0 0 0 0 0 0 0 0 0 0 0 0 0 0 0 0 0 0 0 0 0 0 0 0 0 0 0 0 0 0 0 0 0 0 0 0 0 0 0 0 0 0 0 0 0 0 0 0 0 0 0 0 0 0 0 0 0 0 0 0 0 0 0 0 0 0 0 0 0 0 0 0 0 0 0 0  ].'"  tsamp=2.5  OutMin=[]  OutMax=[]  OutDataTypeStr=double  OutputDataTypeScalingMode=double  OutDataType=fixdt(0,8)  ConRadixGroup=Best Precision: Vector-wise  OutScaling=2^-12
  Repeating Sequence Stair4 : simulink/Sources/Repeating Sequence Stair  Commented=on  OutValues="[0 1 2 3 4 5 6 7 8 9 10 10 10 10 10 10 10 10 10 10 10 10 10 10 10 10 10 10 10 10 10 11 12 13 14 15 16 17 18 19 20 20 20 20 20 20 20 20 20 20 20 19 18 17 16 15 14 13 12 11 10 10 10 10 10 10 10 10 10 10 10 10 10 10 10 10 10 10 10 10 10 10 10 10 10 10 10 10 10 10 10 10 10 10 10 10 10 10 10 10  ].'"  tsamp=2.5  OutMin=[]  OutMax=[]  OutDataTypeStr=double  OutputDataTypeScalingMode=double  OutDataType=fixdt(0,8)  ConRadixGroup=Best Precision: Vector-wise  OutScaling=2^-12
  Repeating Sequence Stair5 : simulink/Sources/Repeating Sequence Stair  Commented=on  OutValues=[0 0 0 0 0 0 0 0 0 0 0 0.5 1 1.5 2 2.5 3 3.5 4 4.5 5 5 5 5 5 5 5 5 5 5 5 5 5 5 5 5 5 5 5 5 5 5.5 6 6.5 7 7.5 8 8.5 9 9.5 10 10 10 10 10 10 10 10 10 10 10 10 10 10 10 10 10 10 10 10 10 10 10 10 10 10 10 10 10 10 10 10 10 10 10 10 10 10 10 10 10 10 10 10 10 10 10 10 10 10 10 10 10 10 10 10 10 10 10 10 10 10 10 10 10 10 10 10 10 10 10 10 10 10 10 10].'  tsamp=2.5  OutMin=[]  OutMax=[]  OutDataTypeStr=double  OutputDataTypeScalingMode=double  OutDataType=fixdt(0,8)  ConRadixGroup=Best Precision: Vector-wise  OutScaling=2^-12
  Repeating Sequence Stair6 : simulink/Sources/Repeating Sequence Stair  Commented=on  OutValues="[0 0 0 0 0 0 0 0 0 0 0 0 0 0 0 0 0 0 0 0 0 1 2 3 4 5 6 7 8 9 10 10 10 10 10 10 10 10 10 10 10 10 10 10 10 10 10 10 10 10 10 10 10 10 10 10 10 10 10 10 10 10 10 10 10 10 10 10 10 10 10 10 10 10 10 10 10 10 10 10 10 10 10 10 10 10 10 10 10 10 10 10 10 10 10 10 10 10 10 10 10 10 10 10 10 10 10 10 10 10 10 10 10 10 10 10 10 10 10 10 10 10 10 10 10 10 10 10 10 10 10 10 10 10  ].'"  tsamp=2.5  OutMin=[]  OutMax=[]  OutDataTypeStr=double  OutputDataTypeScalingMode=double  OutDataType=fixdt(0,8)  ConRadixGroup=Best Precision: Vector-wise  OutScaling=2^-12
  inp : Outport
  wires:
  Mux/1 -> inp/1
  Repeating Sequence Stair3/1 -> Mux/6
  Ground/1 -> Mux/4, Mux/5
  Repeating Sequence Stair13/1 -> Mux/1
  Repeating Sequence Stair14/1 -> Mux/2
  Repeating Sequence Stair15/1 -> Mux/3

== system ANN_and_Fuzzy_NCD/ ANN x 4  1/ANN X ==
  Input : Inport  PortDimensions=2
      mask Display: e = 0.06;c1 = [120 230 180]/255;c2 = ([120 230 180]+0)/(256+128);c3 = ([120 230 180]+128)/(256+128);patch([0 1 1 0],[0 0 1 1],c1);patch([0 1 1 1-e 1-e 0+e],[0 0 1 1-e 0+e 0+e],c2);patch([0 0 1 1-e 0+e 0+e],[0 1 1 1-e 1-e 0+e],c3);plot([0 1 1 0 0],[0 0 1 1 0]);
  Layer 1 : Subsystem
      mask Display: e = 0.06;c1 = [120 150 230]/255;c2 = ([120 150 230]+0)/383;c3 = ([120 150 230]+128)/383;patch([0 1 1 0],[0 0 1 1],c1);patch([0 1 1 1-e 1-e 0+e],[0 0 1 1-e 0+e 0+e],c2);patch([0 0 1 1-e 0+e 0+e],[0 1 1 1-e 1-e 0+e],c3);plot([0 1 1 0 0],[0 0 1 1 0]);
  Layer 2 : Subsystem
      mask Display: e = 0.06;c1 = [120 150 230]/255;c2 = ([120 150 230]+0)/383;c3 = ([120 150 230]+128)/383;patch([0 1 1 0],[0 0 1 1],c1);patch([0 1 1 1-e 1-e 0+e],[0 0 1 1-e 0+e 0+e],c2);patch([0 0 1 1-e 0+e 0+e],[0 1 1 1-e 1-e 0+e],c3);plot([0 1 1 0 0],[0 0 1 1 0]);
  Layer 3 : Subsystem
      mask Display: e = 0.06;c1 = [120 150 230]/255;c2 = ([120 150 230]+0)/383;c3 = ([120 150 230]+128)/383;patch([0 1 1 0],[0 0 1 1],c1);patch([0 1 1 1-e 1-e 0+e],[0 0 1 1-e 0+e 0+e],c2);patch([0 0 1 1-e 0+e 0+e],[0 1 1 1-e 1-e 0+e],c3);plot([0 1 1 0 0],[0 0 1 1 0]);
  Process Input 1 : Subsystem
      mask Display: e = 0.06;c1 = [120 150 230]/255;c2 = ([120 150 230]+0)/383;c3 = ([120 150 230]+128)/383;patch([0 1 1 0],[0 0 1 1],c1);patch([0 1 1 1-e 1-e 0+e],[0 0 1 1-e 0+e 0+e],c2);patch([0 0 1 1-e 0+e 0+e],[0 1 1 1-e 1-e 0+e],c3);plot([0 1 1 0 0],[0 0 1 1 0]);
  Process Output 1 : Subsystem
      mask Display: e = 0.06;c1 = [120 150 230]/255;c2 = ([120 150 230]+0)/383;c3 = ([120 150 230]+128)/383;patch([0 1 1 0],[0 0 1 1],c1);patch([0 1 1 1-e 1-e 0+e],[0 0 1 1-e 0+e 0+e],c2);patch([0 0 1 1-e 0+e 0+e],[0 1 1 1-e 1-e 0+e],c3);plot([0 1 1 0 0],[0 0 1 1 0]);
  Output : Outport  InitialOutput=0
      mask Display: e = 0.06;c1 = [120 230 180]/255;c2 = ([120 230 180]+0)/(256+128);c3 = ([120 230 180]+128)/(256+128);patch([0 1 1 0],[0 0 1 1],c1);patch([0 1 1 1-e 1-e 0+e],[0 0 1 1-e 0+e 0+e],c2);patch([0 0 1 1-e 0+e 0+e],[0 1 1 1-e 1-e 0+e],c3);plot([0 1 1 0 0],[0 0 1 1 0]);
  wires:
  Input/1 -> Process Input 1/1(x)
  Process Output 1/1(y) -> Output/1
  Process Input 1/1(p) -> Layer 1/1("p{1}")
  Layer 1/1("a{1}") -> [feedback1]
  [feedback1] -> Layer 2/1("a{1} ")
  Layer 2/1("a{2}") -> [feedback2]
  [feedback2] -> Layer 3/1("a{2} ")
  Layer 3/1("a{3}") -> Process Output 1/1(a)

== system ANN_and_Fuzzy_NCD/ ANN x 4  1/ANN Y ==
  Input : Inport  PortDimensions=2
      mask Display: e = 0.06;c1 = [120 230 180]/255;c2 = ([120 230 180]+0)/(256+128);c3 = ([120 230 180]+128)/(256+128);patch([0 1 1 0],[0 0 1 1],c1);patch([0 1 1 1-e 1-e 0+e],[0 0 1 1-e 0+e 0+e],c2);patch([0 0 1 1-e 0+e 0+e],[0 1 1 1-e 1-e 0+e],c3);plot([0 1 1 0 0],[0 0 1 1 0]);
  Layer 1 : Subsystem
      mask Display: e = 0.06;c1 = [120 150 230]/255;c2 = ([120 150 230]+0)/383;c3 = ([120 150 230]+128)/383;patch([0 1 1 0],[0 0 1 1],c1);patch([0 1 1 1-e 1-e 0+e],[0 0 1 1-e 0+e 0+e],c2);patch([0 0 1 1-e 0+e 0+e],[0 1 1 1-e 1-e 0+e],c3);plot([0 1 1 0 0],[0 0 1 1 0]);
  Layer 2 : Subsystem
      mask Display: e = 0.06;c1 = [120 150 230]/255;c2 = ([120 150 230]+0)/383;c3 = ([120 150 230]+128)/383;patch([0 1 1 0],[0 0 1 1],c1);patch([0 1 1 1-e 1-e 0+e],[0 0 1 1-e 0+e 0+e],c2);patch([0 0 1 1-e 0+e 0+e],[0 1 1 1-e 1-e 0+e],c3);plot([0 1 1 0 0],[0 0 1 1 0]);
  Layer 3 : Subsystem
      mask Display: e = 0.06;c1 = [120 150 230]/255;c2 = ([120 150 230]+0)/383;c3 = ([120 150 230]+128)/383;patch([0 1 1 0],[0 0 1 1],c1);patch([0 1 1 1-e 1-e 0+e],[0 0 1 1-e 0+e 0+e],c2);patch([0 0 1 1-e 0+e 0+e],[0 1 1 1-e 1-e 0+e],c3);plot([0 1 1 0 0],[0 0 1 1 0]);
  Process Input 1 : Subsystem
      mask Display: e = 0.06;c1 = [120 150 230]/255;c2 = ([120 150 230]+0)/383;c3 = ([120 150 230]+128)/383;patch([0 1 1 0],[0 0 1 1],c1);patch([0 1 1 1-e 1-e 0+e],[0 0 1 1-e 0+e 0+e],c2);patch([0 0 1 1-e 0+e 0+e],[0 1 1 1-e 1-e 0+e],c3);plot([0 1 1 0 0],[0 0 1 1 0]);
  Process Output 1 : Subsystem
      mask Display: e = 0.06;c1 = [120 150 230]/255;c2 = ([120 150 230]+0)/383;c3 = ([120 150 230]+128)/383;patch([0 1 1 0],[0 0 1 1],c1);patch([0 1 1 1-e 1-e 0+e],[0 0 1 1-e 0+e 0+e],c2);patch([0 0 1 1-e 0+e 0+e],[0 1 1 1-e 1-e 0+e],c3);plot([0 1 1 0 0],[0 0 1 1 0]);
  Output : Outport  InitialOutput=0
      mask Display: e = 0.06;c1 = [120 230 180]/255;c2 = ([120 230 180]+0)/(256+128);c3 = ([120 230 180]+128)/(256+128);patch([0 1 1 0],[0 0 1 1],c1);patch([0 1 1 1-e 1-e 0+e],[0 0 1 1-e 0+e 0+e],c2);patch([0 0 1 1-e 0+e 0+e],[0 1 1 1-e 1-e 0+e],c3);plot([0 1 1 0 0],[0 0 1 1 0]);
  wires:
  Input/1 -> Process Input 1/1(x)
  Process Output 1/1(y) -> Output/1
  Process Input 1/1(p) -> Layer 1/1("p{1}")
  Layer 1/1("a{1}") -> [feedback1]
  [feedback1] -> Layer 2/1("a{1} ")
  Layer 2/1("a{2}") -> [feedback2]
  [feedback2] -> Layer 3/1("a{2} ")
  Layer 3/1("a{3}") -> Process Output 1/1(a)

== system ANN_and_Fuzzy_NCD/ ANN x 4  1/ANN Z ==
  Input : Inport  PortDimensions=2
      mask Display: e = 0.06;c1 = [120 230 180]/255;c2 = ([120 230 180]+0)/(256+128);c3 = ([120 230 180]+128)/(256+128);patch([0 1 1 0],[0 0 1 1],c1);patch([0 1 1 1-e 1-e 0+e],[0 0 1 1-e 0+e 0+e],c2);patch([0 0 1 1-e 0+e 0+e],[0 1 1 1-e 1-e 0+e],c3);plot([0 1 1 0 0],[0 0 1 1 0]);
  Layer 1 : Subsystem
      mask Display: e = 0.06;c1 = [120 150 230]/255;c2 = ([120 150 230]+0)/383;c3 = ([120 150 230]+128)/383;patch([0 1 1 0],[0 0 1 1],c1);patch([0 1 1 1-e 1-e 0+e],[0 0 1 1-e 0+e 0+e],c2);patch([0 0 1 1-e 0+e 0+e],[0 1 1 1-e 1-e 0+e],c3);plot([0 1 1 0 0],[0 0 1 1 0]);
  Layer 2 : Subsystem
      mask Display: e = 0.06;c1 = [120 150 230]/255;c2 = ([120 150 230]+0)/383;c3 = ([120 150 230]+128)/383;patch([0 1 1 0],[0 0 1 1],c1);patch([0 1 1 1-e 1-e 0+e],[0 0 1 1-e 0+e 0+e],c2);patch([0 0 1 1-e 0+e 0+e],[0 1 1 1-e 1-e 0+e],c3);plot([0 1 1 0 0],[0 0 1 1 0]);
  Layer 3 : Subsystem
      mask Display: e = 0.06;c1 = [120 150 230]/255;c2 = ([120 150 230]+0)/383;c3 = ([120 150 230]+128)/383;patch([0 1 1 0],[0 0 1 1],c1);patch([0 1 1 1-e 1-e 0+e],[0 0 1 1-e 0+e 0+e],c2);patch([0 0 1 1-e 0+e 0+e],[0 1 1 1-e 1-e 0+e],c3);plot([0 1 1 0 0],[0 0 1 1 0]);
  Process Input 1 : Subsystem
      mask Display: e = 0.06;c1 = [120 150 230]/255;c2 = ([120 150 230]+0)/383;c3 = ([120 150 230]+128)/383;patch([0 1 1 0],[0 0 1 1],c1);patch([0 1 1 1-e 1-e 0+e],[0 0 1 1-e 0+e 0+e],c2);patch([0 0 1 1-e 0+e 0+e],[0 1 1 1-e 1-e 0+e],c3);plot([0 1 1 0 0],[0 0 1 1 0]);
  Process Output 1 : Subsystem
      mask Display: e = 0.06;c1 = [120 150 230]/255;c2 = ([120 150 230]+0)/383;c3 = ([120 150 230]+128)/383;patch([0 1 1 0],[0 0 1 1],c1);patch([0 1 1 1-e 1-e 0+e],[0 0 1 1-e 0+e 0+e],c2);patch([0 0 1 1-e 0+e 0+e],[0 1 1 1-e 1-e 0+e],c3);plot([0 1 1 0 0],[0 0 1 1 0]);
  Output : Outport  InitialOutput=0
      mask Display: e = 0.06;c1 = [120 230 180]/255;c2 = ([120 230 180]+0)/(256+128);c3 = ([120 230 180]+128)/(256+128);patch([0 1 1 0],[0 0 1 1],c1);patch([0 1 1 1-e 1-e 0+e],[0 0 1 1-e 0+e 0+e],c2);patch([0 0 1 1-e 0+e 0+e],[0 1 1 1-e 1-e 0+e],c3);plot([0 1 1 0 0],[0 0 1 1 0]);
  wires:
  Input/1 -> Process Input 1/1(x)
  Process Output 1/1(y) -> Output/1
  Process Input 1/1(p) -> Layer 1/1("p{1}")
  Layer 1/1("a{1}") -> [feedback1]
  [feedback1] -> Layer 2/1("a{1} ")
  Layer 2/1("a{2}") -> [feedback2]
  [feedback2] -> Layer 3/1("a{2} ")
  Layer 3/1("a{3}") -> Process Output 1/1(a)

== system ANN_and_Fuzzy_NCD/ ANN x 4  1/Subsystem ==
  In1 : Inport
  Derivative : Derivative
  Mux : Mux  Inputs=2
  Out1 : Outport
  wires:
  In1/1 -> Mux/1, Derivative/1
  Mux/1 -> Out1/1
  Derivative/1 -> Mux/2

== system ANN_and_Fuzzy_NCD/ ANN x 4  1/Subsystem1 ==
  In1 : Inport
  Derivative : Derivative
  Mux : Mux  Inputs=2
  Out1 : Outport
  wires:
  Derivative/1 -> Mux/2
  In1/1 -> Derivative/1, Mux/1
  Mux/1 -> Out1/1

== system ANN_and_Fuzzy_NCD/ ANN x 4  1/Subsystem2 ==
  In1 : Inport
  Derivative : Derivative
  Mux : Mux  Inputs=2
  Out1 : Outport
  wires:
  Derivative/1 -> Mux/2
  In1/1 -> Derivative/1, Mux/1
  Mux/1 -> Out1/1

== system ANN_and_Fuzzy_NCD/ ANN x 4  1/X_1 ==
  Input : Inport  PortDimensions=2
      mask Display: e = 0.06;c1 = [120 230 180]/255;c2 = ([120 230 180]+0)/(256+128);c3 = ([120 230 180]+128)/(256+128);patch([0 1 1 0],[0 0 1 1],c1);patch([0 1 1 1-e 1-e 0+e],[0 0 1 1-e 0+e 0+e],c2);patch([0 0 1 1-e 0+e 0+e],[0 1 1 1-e 1-e 0+e],c3);plot([0 1 1 0 0],[0 0 1 1 0]);
  Layer 1 : Subsystem
      mask Display: e = 0.06;c1 = [120 150 230]/255;c2 = ([120 150 230]+0)/383;c3 = ([120 150 230]+128)/383;patch([0 1 1 0],[0 0 1 1],c1);patch([0 1 1 1-e 1-e 0+e],[0 0 1 1-e 0+e 0+e],c2);patch([0 0 1 1-e 0+e 0+e],[0 1 1 1-e 1-e 0+e],c3);plot([0 1 1 0 0],[0 0 1 1 0]);
  Layer 2 : Subsystem
      mask Display: e = 0.06;c1 = [120 150 230]/255;c2 = ([120 150 230]+0)/383;c3 = ([120 150 230]+128)/383;patch([0 1 1 0],[0 0 1 1],c1);patch([0 1 1 1-e 1-e 0+e],[0 0 1 1-e 0+e 0+e],c2);patch([0 0 1 1-e 0+e 0+e],[0 1 1 1-e 1-e 0+e],c3);plot([0 1 1 0 0],[0 0 1 1 0]);
  Layer 3 : Subsystem
      mask Display: e = 0.06;c1 = [120 150 230]/255;c2 = ([120 150 230]+0)/383;c3 = ([120 150 230]+128)/383;patch([0 1 1 0],[0 0 1 1],c1);patch([0 1 1 1-e 1-e 0+e],[0 0 1 1-e 0+e 0+e],c2);patch([0 0 1 1-e 0+e 0+e],[0 1 1 1-e 1-e 0+e],c3);plot([0 1 1 0 0],[0 0 1 1 0]);
  Process Input 1 : Subsystem
      mask Display: e = 0.06;c1 = [120 150 230]/255;c2 = ([120 150 230]+0)/383;c3 = ([120 150 230]+128)/383;patch([0 1 1 0],[0 0 1 1],c1);patch([0 1 1 1-e 1-e 0+e],[0 0 1 1-e 0+e 0+e],c2);patch([0 0 1 1-e 0+e 0+e],[0 1 1 1-e 1-e 0+e],c3);plot([0 1 1 0 0],[0 0 1 1 0]);
  Process Output 1 : Subsystem
      mask Display: e = 0.06;c1 = [120 150 230]/255;c2 = ([120 150 230]+0)/383;c3 = ([120 150 230]+128)/383;patch([0 1 1 0],[0 0 1 1],c1);patch([0 1 1 1-e 1-e 0+e],[0 0 1 1-e 0+e 0+e],c2);patch([0 0 1 1-e 0+e 0+e],[0 1 1 1-e 1-e 0+e],c3);plot([0 1 1 0 0],[0 0 1 1 0]);
  Output : Outport  InitialOutput=0
      mask Display: e = 0.06;c1 = [120 230 180]/255;c2 = ([120 230 180]+0)/(256+128);c3 = ([120 230 180]+128)/(256+128);patch([0 1 1 0],[0 0 1 1],c1);patch([0 1 1 1-e 1-e 0+e],[0 0 1 1-e 0+e 0+e],c2);patch([0 0 1 1-e 0+e 0+e],[0 1 1 1-e 1-e 0+e],c3);plot([0 1 1 0 0],[0 0 1 1 0]);
  wires:
  Input/1 -> Process Input 1/1(x)
  Process Output 1/1(y) -> Output/1
  Process Input 1/1(p) -> Layer 1/1("p{1}")
  Layer 1/1("a{1}") -> [feedback1]
  [feedback1] -> Layer 2/1("a{1} ")
  Layer 2/1("a{2}") -> [feedback2]
  [feedback2] -> Layer 3/1("a{2} ")
  Layer 3/1("a{3}") -> Process Output 1/1(a)

== system ANN_and_Fuzzy_NCD/ ANN x 4  1/Y_1 ==
  Input : Inport  PortDimensions=2
      mask Display: e = 0.06;c1 = [120 230 180]/255;c2 = ([120 230 180]+0)/(256+128);c3 = ([120 230 180]+128)/(256+128);patch([0 1 1 0],[0 0 1 1],c1);patch([0 1 1 1-e 1-e 0+e],[0 0 1 1-e 0+e 0+e],c2);patch([0 0 1 1-e 0+e 0+e],[0 1 1 1-e 1-e 0+e],c3);plot([0 1 1 0 0],[0 0 1 1 0]);
  Layer 1 : Subsystem
      mask Display: e = 0.06;c1 = [120 150 230]/255;c2 = ([120 150 230]+0)/383;c3 = ([120 150 230]+128)/383;patch([0 1 1 0],[0 0 1 1],c1);patch([0 1 1 1-e 1-e 0+e],[0 0 1 1-e 0+e 0+e],c2);patch([0 0 1 1-e 0+e 0+e],[0 1 1 1-e 1-e 0+e],c3);plot([0 1 1 0 0],[0 0 1 1 0]);
  Layer 2 : Subsystem
      mask Display: e = 0.06;c1 = [120 150 230]/255;c2 = ([120 150 230]+0)/383;c3 = ([120 150 230]+128)/383;patch([0 1 1 0],[0 0 1 1],c1);patch([0 1 1 1-e 1-e 0+e],[0 0 1 1-e 0+e 0+e],c2);patch([0 0 1 1-e 0+e 0+e],[0 1 1 1-e 1-e 0+e],c3);plot([0 1 1 0 0],[0 0 1 1 0]);
  Layer 3 : Subsystem
      mask Display: e = 0.06;c1 = [120 150 230]/255;c2 = ([120 150 230]+0)/383;c3 = ([120 150 230]+128)/383;patch([0 1 1 0],[0 0 1 1],c1);patch([0 1 1 1-e 1-e 0+e],[0 0 1 1-e 0+e 0+e],c2);patch([0 0 1 1-e 0+e 0+e],[0 1 1 1-e 1-e 0+e],c3);plot([0 1 1 0 0],[0 0 1 1 0]);
  Process Input 1 : Subsystem
      mask Display: e = 0.06;c1 = [120 150 230]/255;c2 = ([120 150 230]+0)/383;c3 = ([120 150 230]+128)/383;patch([0 1 1 0],[0 0 1 1],c1);patch([0 1 1 1-e 1-e 0+e],[0 0 1 1-e 0+e 0+e],c2);patch([0 0 1 1-e 0+e 0+e],[0 1 1 1-e 1-e 0+e],c3);plot([0 1 1 0 0],[0 0 1 1 0]);
  Process Output 1 : Subsystem
      mask Display: e = 0.06;c1 = [120 150 230]/255;c2 = ([120 150 230]+0)/383;c3 = ([120 150 230]+128)/383;patch([0 1 1 0],[0 0 1 1],c1);patch([0 1 1 1-e 1-e 0+e],[0 0 1 1-e 0+e 0+e],c2);patch([0 0 1 1-e 0+e 0+e],[0 1 1 1-e 1-e 0+e],c3);plot([0 1 1 0 0],[0 0 1 1 0]);
  Output : Outport  InitialOutput=0
      mask Display: e = 0.06;c1 = [120 230 180]/255;c2 = ([120 230 180]+0)/(256+128);c3 = ([120 230 180]+128)/(256+128);patch([0 1 1 0],[0 0 1 1],c1);patch([0 1 1 1-e 1-e 0+e],[0 0 1 1-e 0+e 0+e],c2);patch([0 0 1 1-e 0+e 0+e],[0 1 1 1-e 1-e 0+e],c3);plot([0 1 1 0 0],[0 0 1 1 0]);
  wires:
  Input/1 -> Process Input 1/1(x)
  Process Output 1/1(y) -> Output/1
  Process Input 1/1(p) -> Layer 1/1("p{1}")
  Layer 1/1("a{1}") -> [feedback1]
  [feedback1] -> Layer 2/1("a{1} ")
  Layer 2/1("a{2}") -> [feedback2]
  [feedback2] -> Layer 3/1("a{2} ")
  Layer 3/1("a{3}") -> Process Output 1/1(a)

== system ANN_and_Fuzzy_NCD/ ANN x 4  1/Z_1 ==
  Input : Inport  PortDimensions=2
      mask Display: e = 0.06;c1 = [120 230 180]/255;c2 = ([120 230 180]+0)/(256+128);c3 = ([120 230 180]+128)/(256+128);patch([0 1 1 0],[0 0 1 1],c1);patch([0 1 1 1-e 1-e 0+e],[0 0 1 1-e 0+e 0+e],c2);patch([0 0 1 1-e 0+e 0+e],[0 1 1 1-e 1-e 0+e],c3);plot([0 1 1 0 0],[0 0 1 1 0]);
  Layer 1 : Subsystem
      mask Display: e = 0.06;c1 = [120 150 230]/255;c2 = ([120 150 230]+0)/383;c3 = ([120 150 230]+128)/383;patch([0 1 1 0],[0 0 1 1],c1);patch([0 1 1 1-e 1-e 0+e],[0 0 1 1-e 0+e 0+e],c2);patch([0 0 1 1-e 0+e 0+e],[0 1 1 1-e 1-e 0+e],c3);plot([0 1 1 0 0],[0 0 1 1 0]);
  Layer 2 : Subsystem
      mask Display: e = 0.06;c1 = [120 150 230]/255;c2 = ([120 150 230]+0)/383;c3 = ([120 150 230]+128)/383;patch([0 1 1 0],[0 0 1 1],c1);patch([0 1 1 1-e 1-e 0+e],[0 0 1 1-e 0+e 0+e],c2);patch([0 0 1 1-e 0+e 0+e],[0 1 1 1-e 1-e 0+e],c3);plot([0 1 1 0 0],[0 0 1 1 0]);
  Layer 3 : Subsystem
      mask Display: e = 0.06;c1 = [120 150 230]/255;c2 = ([120 150 230]+0)/383;c3 = ([120 150 230]+128)/383;patch([0 1 1 0],[0 0 1 1],c1);patch([0 1 1 1-e 1-e 0+e],[0 0 1 1-e 0+e 0+e],c2);patch([0 0 1 1-e 0+e 0+e],[0 1 1 1-e 1-e 0+e],c3);plot([0 1 1 0 0],[0 0 1 1 0]);
  Process Input 1 : Subsystem
      mask Display: e = 0.06;c1 = [120 150 230]/255;c2 = ([120 150 230]+0)/383;c3 = ([120 150 230]+128)/383;patch([0 1 1 0],[0 0 1 1],c1);patch([0 1 1 1-e 1-e 0+e],[0 0 1 1-e 0+e 0+e],c2);patch([0 0 1 1-e 0+e 0+e],[0 1 1 1-e 1-e 0+e],c3);plot([0 1 1 0 0],[0 0 1 1 0]);
  Process Output 1 : Subsystem
      mask Display: e = 0.06;c1 = [120 150 230]/255;c2 = ([120 150 230]+0)/383;c3 = ([120 150 230]+128)/383;patch([0 1 1 0],[0 0 1 1],c1);patch([0 1 1 1-e 1-e 0+e],[0 0 1 1-e 0+e 0+e],c2);patch([0 0 1 1-e 0+e 0+e],[0 1 1 1-e 1-e 0+e],c3);plot([0 1 1 0 0],[0 0 1 1 0]);
  Output : Outport  InitialOutput=0
      mask Display: e = 0.06;c1 = [120 230 180]/255;c2 = ([120 230 180]+0)/(256+128);c3 = ([120 230 180]+128)/(256+128);patch([0 1 1 0],[0 0 1 1],c1);patch([0 1 1 1-e 1-e 0+e],[0 0 1 1-e 0+e 0+e],c2);patch([0 0 1 1-e 0+e 0+e],[0 1 1 1-e 1-e 0+e],c3);plot([0 1 1 0 0],[0 0 1 1 0]);
  wires:
  Input/1 -> Process Input 1/1(x)
  Process Output 1/1(y) -> Output/1
  Process Input 1/1(p) -> Layer 1/1("p{1}")
  Layer 1/1("a{1}") -> [feedback1]
  [feedback1] -> Layer 2/1("a{1} ")
  Layer 2/1("a{2}") -> [feedback2]
  [feedback2] -> Layer 3/1("a{2} ")
  Layer 3/1("a{3}") -> Process Output 1/1(a)

== system ANN_and_Fuzzy_NCD/ FUZZY x 4  /Subsystem1 ==
  Error : Inport
  Demux : Demux  Outputs=3
  Derivative : Derivative
  Fuzzy Logic Controller : fuzblock/Fuzzy Logic  Controller  FIS='fuzzy2_1.fis'  OutputSampleNumber=101  DataType=double  FuzzifiedInputs=off  RuleFiringStrengths=off  RuleOutputs=off  AggregatedOutputs=off  SimulateUsing=Interpreted execution  OutOfRangeInputValueMessage=warning  NoRuleFiredMessage=warning  EmptyOutputFuzzySetMessage=warning
  Gain : Gain  Gain=1.4
  Mux : Mux  Inputs=2
  Set Kd : Constant  Value=72.83
  Set Ki : Constant  Value=1.76
  Set Kp : Constant  Value=28.69
  Subsystem : Subsystem
  Output : Outport
  wires:
  Set Kp/1 -> Subsystem/4(Set Kp)
  Set Ki/1 -> Subsystem/5(Set Ki)
  Set Kd/1 -> Subsystem/6(Set Kd)
  Error/1 -> Mux/1, Derivative/1, Subsystem/7(Error)
  Derivative/1 -> Mux/2
  Mux/1 -> Fuzzy Logic Controller/1
  Fuzzy Logic Controller/1 -> Gain/1
  Demux/1 -> Subsystem/1(Tuned Kp)
  Demux/2 -> Subsystem/2(Tuned Ki)
  Demux/3 -> Subsystem/3(Tuned Kd)
  Gain/1 -> Demux/1
  Subsystem/1(Outport) -> Output/1

== system ANN_and_Fuzzy_NCD/ FUZZY x 4  /Subsystem5 ==
  Error : Inport
  Demux : Demux  Outputs=3
  Derivative : Derivative
  Fuzzy Logic Controller : fuzblock/Fuzzy Logic  Controller  FIS='fuzzy3_1.fis'  OutputSampleNumber=101  DataType=double  FuzzifiedInputs=off  RuleFiringStrengths=off  RuleOutputs=off  AggregatedOutputs=off  SimulateUsing=Interpreted execution  OutOfRangeInputValueMessage=warning  NoRuleFiredMessage=warning  EmptyOutputFuzzySetMessage=warning
  Gain : Gain  Gain=1.2
  Mux : Mux  Inputs=2
  Set Kd : Constant  Value=61.55
  Set Ki : Constant  Value=1.44
  Set Kp : Constant  Value=21.41
  Subsystem : Subsystem
  Output : Outport
  wires:
  Set Kp/1 -> Subsystem/4(Set Kp)
  Set Ki/1 -> Subsystem/5(Set Ki)
  Set Kd/1 -> Subsystem/6(Set Kd)
  Error/1 -> Mux/1, Derivative/1, Subsystem/7(Error)
  Derivative/1 -> Mux/2
  Mux/1 -> Fuzzy Logic Controller/1
  Demux/1 -> Subsystem/1(Tuned Kp)
  Demux/2 -> Subsystem/2(Tuned Ki)
  Demux/3 -> Subsystem/3(Tuned Kd)
  Gain/1 -> Demux/1
  Fuzzy Logic Controller/1 -> Gain/1
  Subsystem/1(Outport) -> Output/1

== system ANN_and_Fuzzy_NCD/ FUZZY x 4  /Subsystem6 ==
  Error : Inport
  Demux : Demux  Outputs=3
  Derivative : Derivative
  Fuzzy Logic Controller : fuzblock/Fuzzy Logic  Controller  FIS='fuzzy4_1.fis'  OutputSampleNumber=101  DataType=double  FuzzifiedInputs=off  RuleFiringStrengths=off  RuleOutputs=off  AggregatedOutputs=off  SimulateUsing=Interpreted execution  OutOfRangeInputValueMessage=warning  NoRuleFiredMessage=warning  EmptyOutputFuzzySetMessage=warning
  Gain : Gain  Gain=1.4
  Mux : Mux  Inputs=2
  Set Kd : Constant  Value=70.6
  Set Ki : Constant  Value=2
  Set Kp : Constant  Value=44.7
  Subsystem : Subsystem
  Output : Outport
  wires:
  Set Kp/1 -> Subsystem/4(Set Kp)
  Set Ki/1 -> Subsystem/5(Set Ki)
  Set Kd/1 -> Subsystem/6(Set Kd)
  Error/1 -> Mux/1, Derivative/1, Subsystem/7(Error)
  Derivative/1 -> Mux/2
  Mux/1 -> Fuzzy Logic Controller/1
  Demux/1 -> Subsystem/1(Tuned Kp)
  Demux/2 -> Subsystem/2(Tuned Ki)
  Demux/3 -> Subsystem/3(Tuned Kd)
  Fuzzy Logic Controller/1 -> Gain/1
  Gain/1 -> Demux/1
  Subsystem/1(Outport) -> Output/1

== system ANN_and_Fuzzy_NCD/1. Six DOF RRC ROV II/Centripetal & Coriolis ==
  vel : Inport
  Demux : Demux  Outputs=2
      settings: DisplayOption=none
  Mux : Mux  Inputs=2
  Product{1..5} (5 alike) : Product  InputSameDT=on  RndMeth=Zero  SaturateOnIntegerOverflow=on  OutDataTypeStr=Inherit: Same as first input
  Rg : Constant  Value=rg
  Sum : Sum  InputSameDT=on  SaturateOnIntegerOverflow=on  OutDataTypeStr=Inherit: Same as first input
  Sum1 : Sum  InputSameDT=on  SaturateOnIntegerOverflow=on  OutDataTypeStr=Inherit: Same as first input
  inertia(3x3) : Gain  Gain=I*eye(3)+[Xudot 0 0;0 Yvdot 0;0 0 Zwdot]  Multiplication=Matrix(K*u)  SaturateOnIntegerOverflow=on  OutDataTypeStr=Inherit: Same as input  ParamDataTypeStr=Inherit: Same as input
  "mass(3x3) " : Gain  Gain=m*eye(3)+[Xudot 0 0;0 Yvdot 0;0 0 Zwdot]  Multiplication=Matrix(K*u)  SaturateOnIntegerOverflow=on  OutDataTypeStr=Inherit: Same as input  ParamDataTypeStr=Inherit: Same as input
  "mass(3x3) " : Gain  Gain=m*eye(3)+[Xudot 0 0;0 Yvdot 0;0 0 Zwdot]  Multiplication=Matrix(K*u)  SaturateOnIntegerOverflow=on  OutDataTypeStr=Inherit: Same as input  ParamDataTypeStr=Inherit: Same as input
  force : Outport  InitialOutput=0
  wires:
  Product1/1 -> Sum/2
  "mass(3x3) "/1 -> Product2/1
  Product2/1 -> Sum/1
  Rg/1 -> Product3/2, "mass(3x3) "/1
  Product3/1 -> Product4/2
  Product4/1 -> Sum1/1
  Product5/1 -> Product2/2, Sum1/2
  Sum1/1 -> "mass(3x3) "/1
  Demux/2 -> Product5/1, Product3/1, Product4/1, Product1/1, inertia(3x3)/1
  Demux/1 -> Product5/2
  vel/1 -> Demux/1
  inertia(3x3)/1 -> Product1/2
  "mass(3x3) "/1 -> Mux/1
  Sum/1 -> Mux/2
  Mux/1 -> force/1

== system ANN_and_Fuzzy_NCD/1. Six DOF RRC ROV II/Hydrodynamic Damping ==
  vel : Inport
  Add : Sum  Inputs=--
  D linear : Gain  Gain=diag(DL)  SaturateOnIntegerOverflow=on  OutDataTypeStr=Inherit: Same as input  ParamDataTypeStr=Inherit: Same as input
  D quadratic : Gain  Gain=diag(DQ)  SaturateOnIntegerOverflow=on  OutDataTypeStr=Inherit: Same as input  ParamDataTypeStr=Inherit: Same as input
  Product : Product  InputSameDT=on  RndMeth=Zero  SaturateOnIntegerOverflow=on  OutDataTypeStr=Inherit: Same as first input
  |u| : Abs
  damping force : Outport  InitialOutput=0
  wires:
  Product/1 -> D quadratic/1
  D quadratic/1 -> Add/2
  vel/1 -> |u|/1, Product/1, D linear/1
  |u|/1 -> Product/2
  Add/1 -> damping force/1
  D linear/1 -> Add/1
